simulink model "maxExpert"  (R2020a)
settings: Solver=VariableStepAuto  StartTime=0.0  StopTime=0.25  RelTol=1e-3
settings Model: Creator=maxwe  LastModifiedBy=maxwe
settings OptimizationCC: BlockReduction=off  DefaultParameterBehavior=Inlined  BufferReuse=off
settings DebuggingCC: UnderSpecifiedDimensionMsg=warning

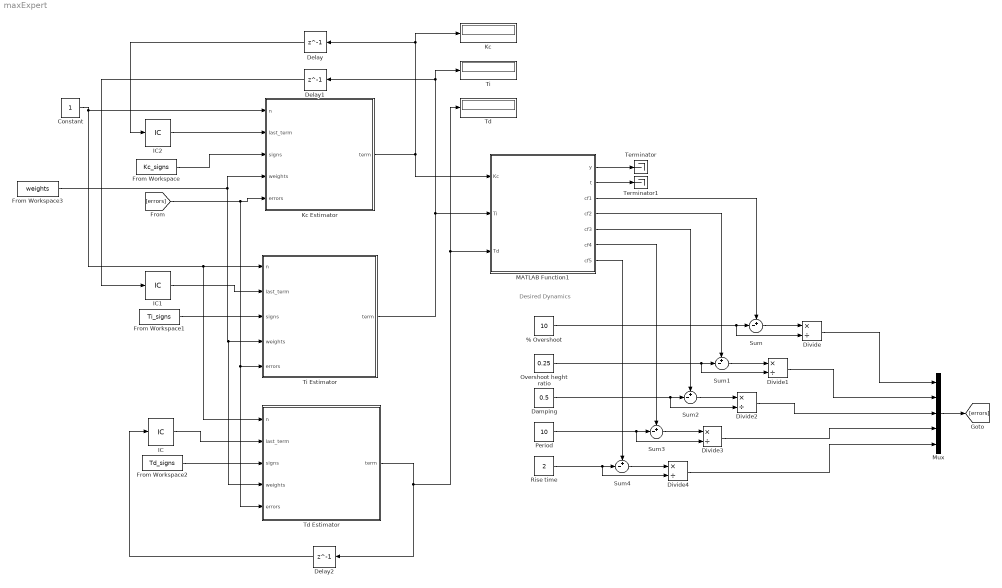
== system maxExpert ==
  note: Desired Dynamics
  % Overshoot : Constant  Value=10
  Constant : Constant
  Damping : Constant  Value=0.5
  Delay : Delay  DelayLength=1  InitialCondition=0
  Delay1 : Delay  DelayLength=1  InitialCondition=0
  Delay2 : Delay  DelayLength=1  InitialCondition=0
  Divide{,1..4} (5 alike) : Product  Inputs=*/
  From Workspace : FromWorkspace  VariableName=Kc_signs
  From Workspace1 : FromWorkspace  VariableName=Ti_signs
  From Workspace2 : FromWorkspace  VariableName=Td_signs
  From Workspace3 : FromWorkspace  VariableName=weights
  IC : InitialCondition  Value=1.69
  IC1 : InitialCondition  Value=6.75
  IC2 : InitialCondition  Value=15
  Kc : Display
  Kc Estimator : MATLAB Function  TreatAsAtomicUnit=on
  MATLAB Function1 : MATLAB Function  TreatAsAtomicUnit=on
  Mux : Mux  Inputs=5
  Overshoot heght ratio : Constant  Value=0.25
  Period : Constant  Value=10
  Rise time : Constant  Value=2
  Sum{,1..4} (5 alike) : Sum  Inputs=+-|
  Td : Display
  Td Estimator : MATLAB Function  TreatAsAtomicUnit=on
  Terminator : Terminator
  Terminator1 : Terminator
  Ti : Display
  Ti Estimator : MATLAB Function  TreatAsAtomicUnit=on
  wires:
  Kc Estimator/1(term) -> Delay/1, Kc/1, MATLAB Function1/1(Kc)
  Ti Estimator/1(term) -> Ti/1, Delay1/1, MATLAB Function1/2(Ti)
  Td Estimator/1(term) -> Delay2/1, Td/1, MATLAB Function1/3(Td)
  Delay2/1 -> IC/1
  IC2/1 -> Kc Estimator/2(last_term)
  IC1/1 -> Ti Estimator/2(last_term)
  IC/1 -> Td Estimator/2(last_term)
  Delay1/1 -> IC1/1
  Delay/1 -> IC2/1
  Constant/1 -> Kc Estimator/1(n), Td Estimator/1(n), Ti Estimator/1(n)
  From Workspace1/1 -> Ti Estimator/3(signs)
  From Workspace2/1 -> Td Estimator/3(signs)
  From Workspace/1 -> Kc Estimator/3(signs)
  From Workspace3/1 -> Kc Estimator/4(weights), Td Estimator/4(weights), Ti Estimator/4(weights)
  % Overshoot/1 -> Divide/2, Sum/2
  Sum/1 -> Divide/1
  MATLAB Function1/3(cf1) -> Sum/1
  Sum1/1 -> Divide1/1
  Overshoot heght ratio/1 -> Divide1/2, Sum1/2
  Sum2/1 -> Divide2/1
  Damping/1 -> Divide2/2, Sum2/2
  Sum3/1 -> Divide3/1
  Period/1 -> Divide3/2, Sum3/2
  Sum4/1 -> Divide4/1
  Rise time/1 -> Divide4/2, Sum4/2
  MATLAB Function1/7(cf5) -> Sum4/1
  MATLAB Function1/6(cf4) -> Sum3/1
  MATLAB Function1/5(cf3) -> Sum2/1
  MATLAB Function1/4(cf2) -> Sum1/1
  Divide/1 -> Mux/1
  Divide1/1 -> Mux/2
  Divide2/1 -> Mux/3
  Divide3/1 -> Mux/4
  Divide4/1 -> Mux/5
  Mux/1 -> [errors]
  [errors] -> Td Estimator/5(errors), Ti Estimator/5(errors), Kc Estimator/5(errors)
  MATLAB Function1/1(y) -> Terminator/1
  MATLAB Function1/2(t) -> Terminator1/1

== matlab function maxExpert/MATLAB Function1 ==
  data: y output; t output; Kc input; Ti input; Td input; cf1 output; cf2 output; cf3 output; cf4 output; cf5 output
function [y,t,cf1,cf2,cf3,cf4,cf5] = fcn(Kc, Ti, Td)
y = 0;
t = 0;
cf1 = 0;
cf2 = 0;
cf3 = 0;
cf4 = 0;
cf5 = 0;

coder.extrinsic('patternExtractor');
[y t cf1 cf2 cf3 cf4 cf5] = patternExtractor(Kc, Ti, Td)

== matlab function maxExpert/Kc Estimator ==
  data: n input; term output; last_term input; signs input; weights input; errors input
function term = termEstimator(n, last_term, signs, weights, errors)
%term = last_term .* (1 + sign((signs .* (weights')) .* errors')/customFibonacci(n));
term = 15;

== matlab function maxExpert/Ti Estimator ==
  data: n input; term output; last_term input; signs input; weights input; errors input
function term = termEstimator(n, last_term, signs, weights, errors)
%term = last_term .* (1 + sign((signs .* (weights')) .* errors')/customFibonacci(n));
term = 5;

== matlab function maxExpert/Td Estimator ==
  data: n input; term output; last_term input; signs input; weights input; errors input
function term = termEstimator(n, last_term, signs, weights, errors)
%[term] = last_term .* (1 + sign((signs .* (weights')) .* errors')/customFibonacci(n));
term = 1.7;
